simulink model "SNAP_Simulink_model_vtest"  (R2020b)
settings: Solver=VariableStepAuto  StartTime=0.0  StopTime=SNAP_sim_length  FixedStep=0.1  MaxStep=10  RelTol=1e-4  EnableMultiTasking=on
InitFcn:
  | SNAP_Simulink_Init_Function
undefined symbols (not defined in the file or in its folder): aeroCIP2006, EN_2BodyModel, EN_Aero, EN_GG, EN_Hyst, EN_Mag, initial_position, initial_velocity, magnitude, SNAP_Br, SNAP_Bs, SNAP_CONST_a3H0, SNAP_CONST_earth_mag_dipole, SNAP_CONST_G_earth, SNAP_CONST_m_earth, SNAP_CONST_mu0, SNAP_CONST_r_earth, SNAP_Hc, SNAP_init_rates, SNAP_JD, SNAP_magnets, SNAP_sat_inertia, SNAP_sat_mass, SNAP_starting_ECI2ECEF_dcm, SNAP_V_hyst, SNAPaero
libraries: vrlib x22, aerolibtransform2 x8, simulink x6, aerolibconvert2 x5, aerolibobsolete x1, aerolibanim x1
(part 1 of 2)
settings Model: Creator=Samir Rawashdeh  LastModifiedBy=colpari
settings DataIOCC: SaveFormat=Array  SignalLoggingSaveFormat=ModelDataLogs  ReturnWorkspaceOutputs=off
settings OptimizationCC: ExpressionDepthLimit=2147483647  LifeSpan=inf
settings DebuggingCC: UnderspecifiedInitializationDetection=Classic  MergeDetectMultiDrivingBlocksExec=none  SolverPrmCheckMsg=warning  MultiTaskCondExecSysMsg=warning  MultiTaskRateTransMsg=warning  SingleTaskRateTransMsg=warning  FcnCallInpInsideContextMsg=warning  StateNameClashWarn=warning  SFUnexpectedBacktrackingDiag=warning  SFNoUnconditionalDefaultTransitionDiag=warning  ArithmeticOperatorsInVariantConditions=warning
settings HardwareCC: ProdBitPerPointer=32  ProdBitPerSizeT=32  ProdBitPerPtrDiffT=32  ProdLargestAtomicFloat=None  ProdIntDivRoundTo=Undefined  ProdEndianess=Unspecified  ProdWordSize=32  ProdHWDeviceType=32-bit Generic
settings ModelReferenceCC: PropagateSignalLabelsOutOfModel=off
settings SFSimCC: SimUseLocalCustomCode=off  CustomCodeUndefinedFunction=UseInterfaceOnly
settings RTWCC: RTWUseLocalCustomCode=off
settings CodeAppCC: StateflowObjectComments=on
settings GRTTargetCC: TargetLangStandard=C89/C90 (ANSI)  CombineOutputUpdateFcns=off  GRTInterface=on
settings ConfigComp: CovMetricSettings=dw  CovSaveCumulativeToWorkspaceVar=on  CovSaveSingleToWorkspaceVar=on  CovExternalEMLEnable=off  CovSFcnEnable=off

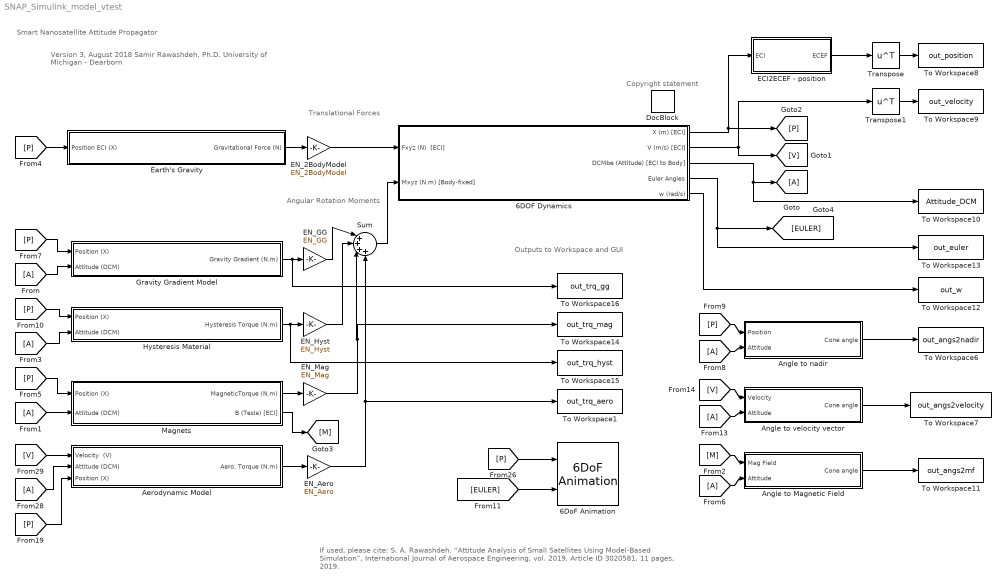
== system SNAP_Simulink_model_vtest ==
  note: If used, please cite:
      | S. A. Rawashdeh. “Attitude Analysis of Small Satellites Using Model-Based Simulation”, International Journal of
      |       Aerospace Engineering, vol. 2019, Article ID 3020581, 11 pages, 2019.
  note: Copyright statement
  note: Smart Nanosatellite Attitude Propagator
  note: Version 3, August 2018
      | Samir Rawashdeh, Ph.D.
      | University of Michigan - Dearborn
  note: Translational Forces
  note: Angular Rotation
      | Moments
  note: Outputs to Workspace and GUI
  "6DOF Dynamics " : Subsystem
  6DoF Animation : aerolibanim/6DoF Animation  u1=[-4000 4000 -2000 2000 -5000 -3000]  u2=10  u3=1000000*4  u4=[0 0 0]  u5=Fixed position  u6=[ 1 1 1 ] * 40000000  u7=15  u8=on
  Aerodynamic Model : Subsystem
  Angle to Magnetic Field : Subsystem
  Angle to nadir : Subsystem
  Angle to velocity vector : Subsystem
  DocBlock : simulink/Model-Wide Utilities/DocBlock  DocumentType=Text
      content=|
      | % See "help.txt" for documentation. More info in can be found at:
      | % sar-lab.net/snap
      | %
      | % -----------------------------------------------------------------------------
      | %   Copyright (c) 2010-2018 Samir A. Rawashdeh
      | %   Electrical and Computer Engineering
      | %   University of Michigan - Dearborn
      | %
      | %   All rights reserved.
      | %
      | %   Redistribution and use in source and binary forms, with or without
      | %   modification, are permitted provided that the following conditions are
      | %   met:
      | %
      | %       * Redistributions of source code must retain the above copyright
      | %         notice, this list of conditions and the following disclaimer.
      | %       * Redistributions in binary form must reproduce the above copyright
      | %         notice, this list of conditions and the following disclaimer in
      | %         the documentation and/or other materials provided with the distribution
      | %
      | %   THIS SOFTWARE IS PROVIDED BY THE COPYRIGHT HOLDERS AND CONTRIBUTORS "AS IS"
      | %   AND ANY EXPRESS OR IMPLIED WARRANTIES, INCLUDING, BUT NOT LIMITED TO, THE
      | %   IMPLIED WARRANTIES OF MERCHANTABILITY AND FITNESS FOR A PARTICULAR PURPOSE
      | %   ARE DISCLAIMED. IN NO EVENT SHALL THE COPYRIGHT OWNER OR CONTRIBUTORS BE
      | %   LIABLE FOR ANY DIRECT, INDIRECT, INCIDENTAL, SPECIAL, EXEMPLARY, OR
      | %   CONSEQUENTIAL DAMAGES (INCLUDING, BUT NOT LIMITED TO, PROCUREMENT OF
      | %   SUBSTITUTE GOODS OR SERVICES; LOSS OF USE, DATA, OR PROFITS; OR BUSINESS
      | %   INTERRUPTION) HOWEVER CAUSED AND ON ANY THEORY OF LIABILITY, WHETHER IN
      | %   CONTRACT, STRICT LIABILITY, OR TORT (INCLUDING NEGLIGENCE OR OTHERWISE)
      | %   ARISING IN ANY WAY OUT OF THE USE OF THIS SOFTWARE, EVEN IF ADVISED OF THE
      | %   POSSIBILITY OF SUCH DAMAGE.
      | %
      | % ----------------------------------------------------------------------------
  ECI2ECEF - position : Subsystem
  EN_2BodyModel : Gain  Gain=EN_2BodyModel
  "EN_Aero " : Gain  Gain=EN_Aero
  EN_GG : Gain  Gain=EN_GG
  EN_Hyst : Gain  Gain=EN_Hyst
  EN_Mag : Gain  Gain=EN_Mag
  Earth's Gravity : Subsystem
  Gravity Gradient Model : Subsystem
  Hysteresis Material : Subsystem
  Magnets : Subsystem
  Sum : Sum  Inputs=|++++
  To Workspace1 : ToWorkspace  VariableName=out_trq_aero  SaveFormat=Structure With Time  SampleTime=-1
  To Workspace10 : ToWorkspace  VariableName=Attitude_DCM  SaveFormat=Structure With Time  SampleTime=-1
  To Workspace11 : ToWorkspace  VariableName=out_angs2mf  SaveFormat=Structure With Time  SampleTime=-1
  To Workspace12 : ToWorkspace  VariableName=out_w  SaveFormat=Structure With Time  SampleTime=-1
  To Workspace13 : ToWorkspace  VariableName=out_euler  SaveFormat=Structure With Time  SampleTime=-1
  To Workspace14 : ToWorkspace  VariableName=out_trq_mag  SaveFormat=Structure With Time  SampleTime=-1
  To Workspace15 : ToWorkspace  VariableName=out_trq_hyst  SaveFormat=Structure With Time  SampleTime=-1
  To Workspace16 : ToWorkspace  VariableName=out_trq_gg  SaveFormat=Structure With Time  SampleTime=-1
  To Workspace6 : ToWorkspace  VariableName=out_angs2nadir  SaveFormat=Structure With Time  SampleTime=-1
  To Workspace7 : ToWorkspace  VariableName=out_angs2velocity  SaveFormat=Structure With Time  SampleTime=-1
  To Workspace8 : ToWorkspace  VariableName=out_position  SaveFormat=Structure With Time  SampleTime=-1
  To Workspace9 : ToWorkspace  VariableName=out_velocity  SaveFormat=Structure With Time  SampleTime=-1
  Transpose : Math  Operator=transpose  SignedPower=on  SaturateOnIntegerOverflow=on
  Transpose1 : Math  Operator=transpose  SignedPower=on  SaturateOnIntegerOverflow=on
  wires:
  Transpose/1 -> To Workspace8/1
  Transpose1/1 -> To Workspace9/1
  "6DOF Dynamics "/3(DCMbe (Attitude) [ECI to Body]) -> To Workspace10/1, [A]
  "6DOF Dynamics "/4(Euler Angles) -> [EULER], To Workspace13/1
  "6DOF Dynamics "/5(w (rad/s)) -> To Workspace12/1
  Gravity Gradient Model/1(Gravity Gradient (N.m)) -> To Workspace16/1, EN_GG/1
  Hysteresis Material/1(Hysteresis Torque (N.m)) -> EN_Hyst/1, To Workspace15/1
  EN_Mag/1 -> Sum/3, To Workspace14/1
  Angle to nadir/1(Cone angle) -> To Workspace6/1
  Angle to velocity vector/1(Cone angle) -> To Workspace7/1
  [P] -> Earth's Gravity/1(Position ECI (X))
  "6DOF Dynamics "/1(X (m) [ECI]) -> ECI2ECEF - position/1(ECI), [P]
  "6DOF Dynamics "/2(V (m/s) [ECI]) -> Transpose1/1, [V]
  [P] -> Gravity Gradient Model/1(Position (X))
  [A] -> Gravity Gradient Model/2(Attitude (DCM))
  [P] -> Magnets/1(Position (X))
  [A] -> Magnets/2(Attitude (DCM))
  Magnets/1(MagneticTorque (N.m)) -> EN_Mag/1
  [A] -> Angle to nadir/2(Attitude)
  [P] -> Angle to nadir/1(Position)
  [A] -> Angle to velocity vector/2(Attitude)
  [V] -> Angle to velocity vector/1(Velocity)
  ECI2ECEF - position/1(ECEF) -> Transpose/1
  Magnets/2(B (Tesla) [ECI]) -> [M]
  Earth's Gravity/1(Gravitational Force (N)) -> EN_2BodyModel/1
  [A] -> Angle to Magnetic Field/2(Attitude)
  Angle to Magnetic Field/1(Cone angle) -> To Workspace11/1
  [M] -> Angle to Magnetic Field/1(Mag Field)
  EN_GG/1 -> Sum/1
  EN_Hyst/1 -> Sum/2
  [V] -> Aerodynamic Model/1(Velocity  (V))
  [A] -> Aerodynamic Model/2(Attitude (DCM))
  [P] -> Aerodynamic Model/3(Position (X))
  [P] -> 6DoF Animation/1
  EN_2BodyModel/1 -> "6DOF Dynamics "/1(Fxyz (N)  [ECI])
  Sum/1 -> "6DOF Dynamics "/2(Mxyz (N.m) [Body-fixed])
  [P] -> Hysteresis Material/1(Position (X))
  [A] -> Hysteresis Material/2(Attitude (DCM))
  Aerodynamic Model/1(Aero. Torque (N.m)) -> "EN_Aero "/1
  "EN_Aero "/1 -> Sum/4, To Workspace1/1
  [EULER] -> 6DoF Animation/2

== system SNAP_Simulink_model_vtest/6DOF Dynamics  ==
  Fxyz (N)  [ECI] : Inport
  Mxyz (N.m) [Body-fixed] : Inport  Port=2
  Rotations - 6DoF (Quaternion) : aerolibobsolete/6DoF (Euler Angles)  units=Metric (MKS)  mtype=Fixed  rep=Quaternion  xme_0=[0 0 0] % not used  Vm_0=[0 0 0] % not used  eul_0=[0 0 0] %[0 pi/1.1 0]  pm_0=SNAP_init_rates %(ones(1,3)*0.5-rand(1,3) )* 2 * .3 *pi/180;  mass_0=SNAP_sat_mass  mass_e=0  mass_f=0  inertia=SNAP_sat_inertia  inertia_e=eye(3)  inertia_f=eye(3)  k_quat=1.0
      settings: SourceProductBaseCode=AE
  Terminator{,1..3,5} (5 alike) : Terminator
  Translation : Subsystem
  zero : Constant  Value=[0 0 0]
  X (m) [ECI] : Outport
  V (m/s) [ECI] : Outport  Port=2
  DCMbe (Attitude) [ECI to Body] : Outport  Port=3
  Euler Angles : Outport  Port=4
  w (rad/s) : Outport  Port=5
  wires:
  Rotations - 6DoF (Quaternion)/2 -> Terminator/1
  Rotations - 6DoF (Quaternion)/1 -> Terminator2/1
  Rotations - 6DoF (Quaternion)/5 -> Terminator1/1
  Translation/1(Xe(m) (ECI)) -> X (m) [ECI]/1
  Translation/2(Ve(m/s) (ECI)) -> V (m/s) [ECI]/1
  Rotations - 6DoF (Quaternion)/6 -> w (rad/s)/1
  Rotations - 6DoF (Quaternion)/8 -> Terminator5/1
  Rotations - 6DoF (Quaternion)/7 -> Terminator3/1
  zero/1 -> Rotations - 6DoF (Quaternion)/1
  Fxyz (N)  [ECI]/1 -> Translation/1(Fxyz (N) (inECI))
  Mxyz (N.m) [Body-fixed]/1 -> Rotations - 6DoF (Quaternion)/2
  Rotations - 6DoF (Quaternion)/3 -> Euler Angles/1
  Rotations - 6DoF (Quaternion)/4 -> DCMbe (Attitude) [ECI to Body]/1

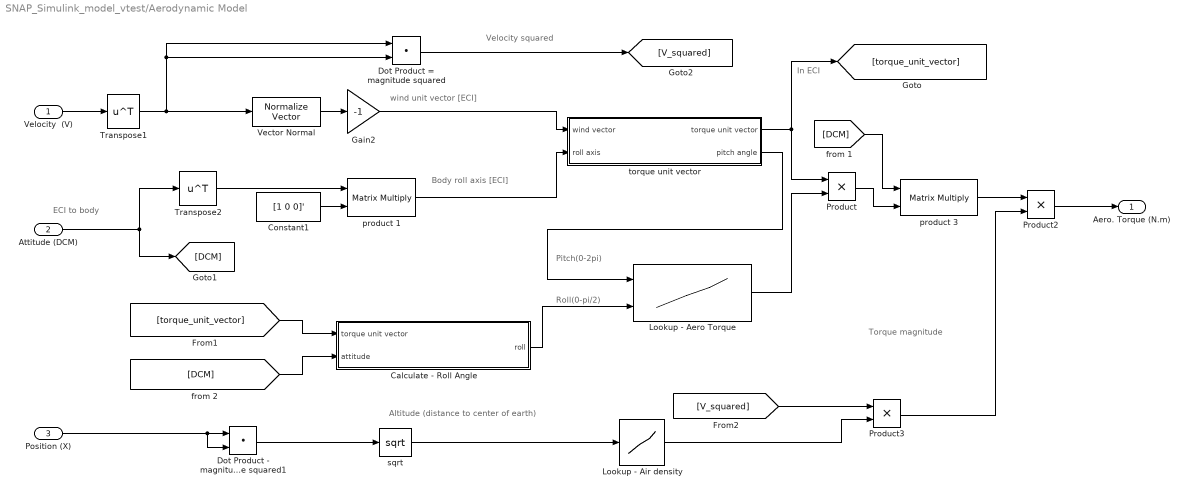
== system SNAP_Simulink_model_vtest/Aerodynamic Model ==
  note: Pitch(0-2pi)
  note: wind unit vector [ECI]
  note: Torque magnitude
  note: Body roll axis [ECI]
  note: In ECI
  note: ECI to body
  note: Velocity squared
  note: Roll(0-pi/2)
  note: Altitude (distance to center of earth)
  Velocity  (V) : Inport
  Attitude (DCM) : Inport  Port=2
  Position (X) : Inport  Port=3
  Calculate - Roll Angle : Subsystem
  Constant1 : Constant  Value=[1 0 0]'
  Dot Product - magnitude squared1 : DotProduct  InputSameDT=on  OutDataTypeStr=Inherit: Inherit via internal rule
  Dot Product = magnitude squared : DotProduct  InputSameDT=on  OutDataTypeStr=Inherit: Inherit via internal rule
  Gain2 : Gain  Gain=-1
  Lookup - Aero Torque : Lookup2D  RowIndex=SNAPaero.pitch  ColumnIndex=SNAPaero.roll  Table=SNAPaero.T
  Lookup - Air density : Lookup  InputValues=SNAPaero.alt_range*1000 + SNAP_CONST_r_earth  Table=SNAPaero.av_density_vs_alt
  Product : Product  RndMeth=Zero
  Product2 : Product  RndMeth=Zero
  Product3 : Product  RndMeth=Zero
  Transpose1 : Math  Operator=transpose  SignedPower=on  SaturateOnIntegerOverflow=on
  Transpose2 : Math  Operator=transpose  SignedPower=on  SaturateOnIntegerOverflow=on
  Vector Normal : vrlib/Utilities/Normalize Vector  maxzero=0
  product 1 : Product  Multiplication=Matrix(*)  RndMeth=Zero
  product 3 : Product  Multiplication=Matrix(*)  RndMeth=Zero
  sqrt : Math  Operator=sqrt  SignedPower=on  SaturateOnIntegerOverflow=on
  torque unit vector : Subsystem
  Aero. Torque (N.m) : Outport
  wires:
  Velocity  (V)/1 -> Transpose1/1
  Dot Product = magnitude squared/1 -> [V_squared]
  Vector Normal/1 -> Gain2/1
  Gain2/1 -> torque unit vector/1(wind vector)
  product 1/1 -> torque unit vector/2(roll axis)
  torque unit vector/1(torque unit vector) -> Product/1, [torque_unit_vector]
  Lookup - Aero Torque/1 -> Product/2
  [DCM] -> product 3/1
  Transpose1/1 -> Vector Normal/1, Dot Product = magnitude squared/2, Dot Product = magnitude squared/1
  Constant1/1 -> product 1/2
  Attitude (DCM)/1 -> [DCM], Transpose2/1
  Product/1 -> product 3/2
  Calculate - Roll Angle/1(roll) -> Lookup - Aero Torque/2
  torque unit vector/2(pitch angle) -> Lookup - Aero Torque/1
  Transpose2/1 -> product 1/1
  [torque_unit_vector] -> Calculate - Roll Angle/1(torque unit vector)
  [DCM] -> Calculate - Roll Angle/2(attitude)
  Position (X)/1 -> Dot Product - magnitude squared1/1, Dot Product - magnitude squared1/2
  Dot Product - magnitude squared1/1 -> sqrt/1
  sqrt/1 -> Lookup - Air density/1
  Lookup - Air density/1 -> Product3/2
  Product3/1 -> Product2/2
  [V_squared] -> Product3/1
  Product2/1 -> Aero. Torque (N.m)/1
  product 3/1 -> Product2/1

== system SNAP_Simulink_model_vtest/Angle to Magnetic Field ==
  note: velocity vector
  Mag Field : Inport
  Attitude : Inport  Port=2
  Normalize Vector : vrlib/Utilities/Normalize Vector  maxzero=0
  cosines to body axes : Subsystem
  Cone angle : Outport
  wires:
  Mag Field/1 -> Normalize Vector/1
  Attitude/1 -> cosines to body axes/2(Attitude)
  cosines to body axes/1(Cone Angles) -> Cone angle/1
  Normalize Vector/1 -> cosines to body axes/1(Reference Vector)

== system SNAP_Simulink_model_vtest/Angle to nadir ==
  note: vector from satellite to earth (nadir)
  Position : Inport
  Attitude : Inport  Port=2
  Gain2 : Gain  Gain=-1
  Normalize Vector : vrlib/Utilities/Normalize Vector  maxzero=0
  cosines to body axes : Subsystem
  Cone angle : Outport
  wires:
  Normalize Vector/1 -> Gain2/1
  Position/1 -> Normalize Vector/1
  cosines to body axes/1(Cone Angles) -> Cone angle/1
  Gain2/1 -> cosines to body axes/1(Reference Vector)
  Attitude/1 -> cosines to body axes/2(Attitude)

== system SNAP_Simulink_model_vtest/Angle to velocity vector ==
  note: velocity vector
  Velocity : Inport
  Attitude : Inport  Port=2
  Normalize Vector : vrlib/Utilities/Normalize Vector  maxzero=0
  cosines to body axes : Subsystem
  Cone angle : Outport
  wires:
  Velocity/1 -> Normalize Vector/1
  Attitude/1 -> cosines to body axes/2(Attitude)
  cosines to body axes/1(Cone Angles) -> Cone angle/1
  Normalize Vector/1 -> cosines to body axes/1(Reference Vector)

== system SNAP_Simulink_model_vtest/ECI2ECEF - position ==
  ECI : Inport
  Constant : Constant  Value=[0 0]
  Constant1 : Constant  Commented=on  Value=SNAP_JD
  Constant2 : Constant  Value=SNAP_starting_ECI2ECEF_dcm
  Direction Cosine Matrix ECI to ECEF1 : Subsystem  Commented=on  AncestorBlock=aerolibtransform2/Direction Cosine Matrix ECI to ECEF  mask{red=IAU-2000/2006, deltaT=Sec, errorflag=Error, extraparamflag=off}
      mask prompts: red "aeroblks:aeroblktransform:blockDCMECItoECEFParamReduction"; deltaT "aeroblks:aeroblktransform:blockDCMECItoECEFParamTimeincrement"; errorflag "aeroblks:aeroblktransform:blockDCMECItoECEFParamActionforoutofrangeinput"; extraparamflag "aeroblks:aeroblktransform:blockDCMECItoECEFParamHigheraccuracyparameters"
      settings: AttributesFormatString=%<red>
      mask TypeOptions red: aeroblks:aeroblktransform:blockDCMECItoECEFParamComboIAU76FK5 | aeroblks:aeroblktransform:blockDCMECItoECEFParamComboIAU20002006
      mask TypeOptions deltaT: aeroblks:aeroblktransform:blockDCMECItoECEFParamComboNone | aeroblks:aeroblktransform:blockDCMECItoECEFParamComboDay | aeroblks:aeroblktransform:blockDCMECItoECEFParamComboHour | aeroblks:aeroblktransform:blockDCMECItoECEFParamComboMin | aeroblks:aeroblktransform:blockDCMECItoECEFParamComboSec
      mask TypeOptions errorflag: aeroblks:aeroblktransform:blockDCMECItoECEFParamComboNone | aeroblks:aeroblktransform:blockDCMECItoECEFParamComboWarning | aeroblks:aeroblktransform:blockDCMECItoECEFParamComboError
      mask Display:
      | port_label('output',1,'DCM_{fi}','texmode','on')
      | port_label('input',1,'JD')
  Gain : Gain  Gain=-1
  Mux : Mux  Inputs=2
  Ramp1 : simulink/Sources/Ramp  slope="7.292115856e-5   %2*pi/(24*60*60)  %radians/second (one rotation per day )"  start=0  X0=0
  Rotation Angles to Direction Cosine Matrix : aerolibtransform2/Rotation Angles to Direction Cosine Matrix  rotationOrder=ZYX
      settings: SourceProductBaseCode=AE
  product 1 : Product  Multiplication=Matrix(*)  RndMeth=Zero
  product 2 : Product  Multiplication=Matrix(*)  RndMeth=Zero
  ECEF : Outport
  wires:
  product 2/1 -> ECEF/1
  ECI/1 -> product 2/1
  Constant1/1 -> Direction Cosine Matrix ECI to ECEF1/1(JD)
  Ramp1/1 -> Gain/1
  Gain/1 -> Mux/1
  Mux/1 -> Rotation Angles to Direction Cosine Matrix/1
  Constant/1 -> Mux/2
  product 1/1 -> product 2/2
  Rotation Angles to Direction Cosine Matrix/1 -> product 1/2
  Constant2/1 -> product 1/1

== system SNAP_Simulink_model_vtest/Earth's Gravity ==
  note: Gravitational
      | acceleration vector
  note: magnitude of acceleration due to gravity
  note: Unit vector towards Nadir
  note: a_gravity = G*m/r^2
  Position ECI (X) : Inport
  Constant : Constant  Value=SNAP_CONST_r_earth
  Divide : Product  Inputs=*/
  Gain1 : Gain  Gain=-1
  Gain2 : Gain  Gain=SNAP_sat_mass
  Gravitational Constant : Constant  Value=SNAP_CONST_m_earth*SNAP_CONST_G_earth
  Math Function : Math  Operator=sqrt  SignedPower=on  SaturateOnIntegerOverflow=on
  Product : Product  RndMeth=Zero
  Scope4 : Scope
  Sum : Sum  Inputs=|+-
  Vector Dot Product = magnitude squared : DotProduct  InputSameDT=on  OutDataTypeStr=Inherit: Inherit via internal rule
  Vector Normal : vrlib/Utilities/Normalize Vector  maxzero=0
  Gravitational Force (N) : Outport
  wires:
  Position ECI (X)/1 -> Vector Normal/1, Vector Dot Product = magnitude squared/1, Vector Dot Product = magnitude squared/2
  Vector Normal/1 -> Gain1/1
  Gain1/1 -> Product/1
  Product/1 -> Gain2/1
  Vector Dot Product = magnitude squared/1 -> Divide/2, Math Function/1
  Divide/1 -> Product/2
  Gravitational Constant/1 -> Divide/1
  Gain2/1 -> Gravitational Force (N)/1
  Math Function/1 -> Sum/1
  Sum/1 -> Scope4/1
  Constant/1 -> Sum/2

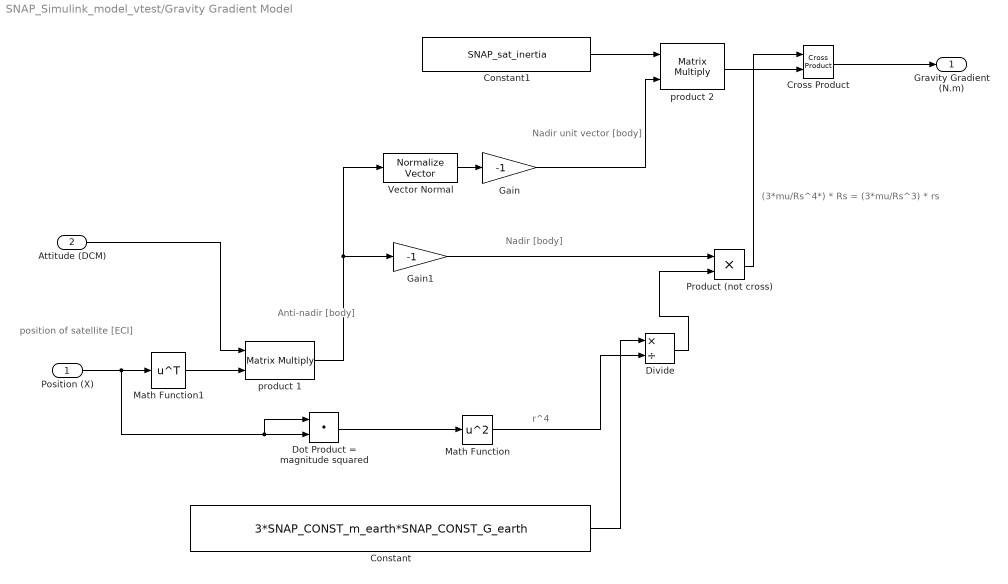
== system SNAP_Simulink_model_vtest/Gravity Gradient Model ==
  note: (3*mu/Rs^4*) * Rs = (3*mu/Rs^3) * rs
  note: Nadir [body]
  note: position of satellite [ECI]
  note: Nadir unit vector
      | [body]
  note: Anti-nadir [body]
  note: r^4
  Position (X) : Inport
  Attitude (DCM) : Inport  Port=2
  Constant : Constant  Value=3*SNAP_CONST_m_earth*SNAP_CONST_G_earth
  Constant1 : Constant  Value=SNAP_sat_inertia
  Cross Product : vrlib/Utilities/Cross Product
  Divide : Product  Inputs=*/
  Dot Product = magnitude squared : DotProduct  InputSameDT=on  OutDataTypeStr=Inherit: Inherit via internal rule
  Gain : Gain  Gain=-1
  Gain1 : Gain  Gain=-1
  Math Function : Math  Operator=square  SignedPower=on  SaturateOnIntegerOverflow=on
  Math Function1 : Math  Operator=transpose  SignedPower=on  SaturateOnIntegerOverflow=on
  Product (not cross) : Product  RndMeth=Zero
  Vector Normal : vrlib/Utilities/Normalize Vector  maxzero=0
  product 1 : Product  Multiplication=Matrix(*)  RndMeth=Zero
  product 2 : Product  Multiplication=Matrix(*)  RndMeth=Zero
  Gravity Gradient (N.m) : Outport
  wires:
  Product (not cross)/1 -> Cross Product/1
  Divide/1 -> Product (not cross)/2
  Constant/1 -> Divide/1
  Math Function/1 -> Divide/2
  Vector Normal/1 -> Gain/1
  Cross Product/1 -> Gravity Gradient (N.m)/1
  Dot Product = magnitude squared/1 -> Math Function/1
  Gain/1 -> product 2/2
  product 2/1 -> Cross Product/2
  Constant1/1 -> product 2/1
  Position (X)/1 -> Dot Product = magnitude squared/2, Dot Product = magnitude squared/1, Math Function1/1
  Attitude (DCM)/1 -> product 1/1
  product 1/1 -> Vector Normal/1, Gain1/1
  Gain1/1 -> Product (not cross)/1
  Math Function1/1 -> product 1/2

== system SNAP_Simulink_model_vtest/Hysteresis Material ==
  note: ECI to Body
  note: T = m X B
  note: B_earth
  note: B_earth [body]
  note: m [body]
  Position (X) : Inport
  Attitude (DCM) : Inport  Port=2
  Cross Product : vrlib/Utilities/Cross Product
  Eearth L-Shell Magnetic Model : Subsystem
  Gain : Gain  Gain=1/SNAP_CONST_mu0
  Hysteresis Curve Model : Subsystem
  Product : Product  Multiplication=Matrix(*)  RndMeth=Zero
  Transpose : Math  Operator=transpose  SignedPower=on  SaturateOnIntegerOverflow=on
  m = B*V/mu0 : Product  RndMeth=Zero
  zero : Constant  Value=SNAP_V_hyst/SNAP_CONST_mu0
  Hysteresis Torque (N.m) : Outport
  wires:
  Product/1 -> Gain/1, Cross Product/2
  Cross Product/1 -> Hysteresis Torque (N.m)/1
  zero/1 -> m = B*V/mu0/2
  m = B*V/mu0/1 -> Cross Product/1
  Attitude (DCM)/1 -> Product/1
  Eearth L-Shell Magnetic Model/1(B (Tesla) in ECI) -> Transpose/1
  Transpose/1 -> Product/2
  Gain/1 -> Hysteresis Curve Model/1(H)
  Hysteresis Curve Model/1(B) -> m = B*V/mu0/1
  Position (X)/1 -> Eearth L-Shell Magnetic Model/1(Position in ECI)

== system SNAP_Simulink_model_vtest/Magnets ==
  note: T = m X B
  note: B_earth [body]
  note: ECI to Body
  Position (X) : Inport
  Attitude (DCM) : Inport  Port=2
  Cross Product : vrlib/Utilities/Cross Product
  Eearth L-Shell Magnetic Model : Subsystem
  Product : Product  Multiplication=Matrix(*)  RndMeth=Zero
  Transpose : Math  Operator=transpose  SignedPower=on  SaturateOnIntegerOverflow=on
  constant : Constant  Value=SNAP_magnets
  MagneticTorque (N.m) : Outport
  B (Tesla) [ECI] : Outport  Port=2
  wires:
  Position (X)/1 -> Eearth L-Shell Magnetic Model/1(Position in ECI)
  Product/1 -> Cross Product/2
  Cross Product/1 -> MagneticTorque (N.m)/1
  constant/1 -> Cross Product/1
  Attitude (DCM)/1 -> Product/1
  Eearth L-Shell Magnetic Model/1(B (Tesla) in ECI) -> Transpose/1, B (Tesla) [ECI]/1
  Transpose/1 -> Product/2

== system SNAP_Simulink_model_vtest/6DOF Dynamics /Translation ==
  note: Force
  note: Acceleration
  note: Velocity
  note: Position
  Fxyz (N) (inECI) : Inport
  Gain : Gain  Gain=1/SNAP_sat_mass
  Integrator : Integrator  InitialCondition=initial_velocity
  Integrator1 : Integrator  InitialCondition=initial_position
  Xe(m) (ECI) : Outport
  Ve(m/s) (ECI) : Outport  Port=2
  wires:
  Fxyz (N) (inECI)/1 -> Gain/1
  Gain/1 -> Integrator/1
  Integrator/1 -> Integrator1/1, Ve(m/s) (ECI)/1
  Integrator1/1 -> Xe(m) (ECI)/1

== system SNAP_Simulink_model_vtest/Aerodynamic Model/Calculate - Roll Angle ==
  note: pitch axis in ECI
  note: Roll(0-pi/2)
  torque unit vector : Inport
  attitude : Inport  Port=2
  Constant2 : Constant  Value=[0 1 0]'
  Constant3 : Constant  Value=pi/2
  Dot Product : DotProduct  InputSameDT=on  OutDataTypeStr=Inherit: Inherit via internal rule
  Modulus : Math  Operator=mod  SignedPower=on  SaturateOnIntegerOverflow=on
  Trigonometric Function1 : Trigonometry  Operator=acos
  product 2 : Product  Multiplication=Matrix(*)  RndMeth=Zero
  roll : Outport
  wires:
  torque unit vector/1 -> Dot Product/1
  product 2/1 -> Dot Product/2
  Dot Product/1 -> Trigonometric Function1/1
  Trigonometric Function1/1 -> Modulus/1
  Constant3/1 -> Modulus/2
  Modulus/1 -> roll/1
  Constant2/1 -> product 2/2
  attitude/1 -> product 2/1

== system SNAP_Simulink_model_vtest/Aerodynamic Model/torque unit vector ==
  wind vector : Inport
  roll axis : Inport  Port=2
  Cross Product : vrlib/Utilities/Cross Product
  Dot Product : DotProduct  InputSameDT=on  OutDataTypeStr=Inherit: Inherit via internal rule
  Normalize Vector : vrlib/Utilities/Normalize Vector  maxzero=0
  Trigonometric Function2 : Trigonometry  Operator=acos
  torque unit vector : Outport
  pitch angle : Outport  Port=2
  wires:
  Normalize Vector/1 -> torque unit vector/1
  Cross Product/1 -> Normalize Vector/1
  wind vector/1 -> Cross Product/1, Dot Product/1
  roll axis/1 -> Cross Product/2, Dot Product/2
  Dot Product/1 -> Trigonometric Function2/1
  Trigonometric Function2/1 -> pitch angle/1

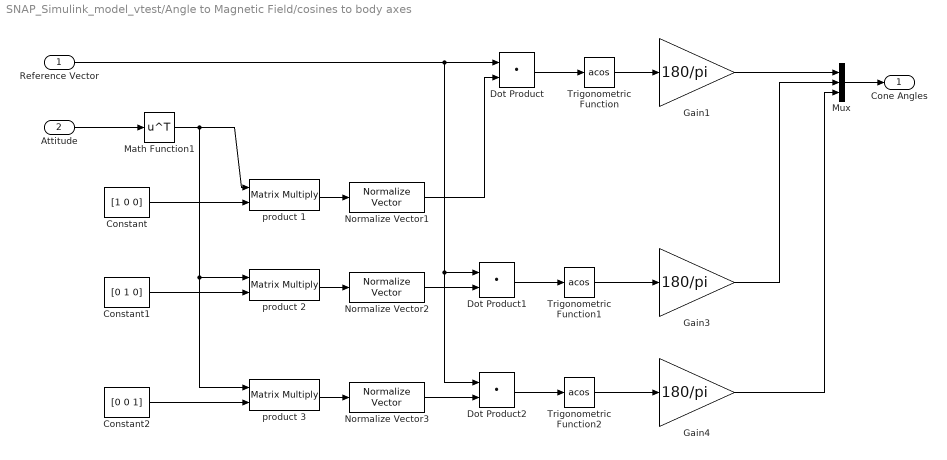
== system SNAP_Simulink_model_vtest/Angle to Magnetic Field/cosines to body axes ==
  Reference Vector : Inport
  Attitude : Inport  Port=2
  Constant : Constant  Value=[1 0 0]
  Constant1 : Constant  Value=[0 1 0]
  Constant2 : Constant  Value=[0 0 1]
  Dot Product : DotProduct  InputSameDT=on  OutDataTypeStr=Inherit: Inherit via internal rule
  Dot Product1 : DotProduct  InputSameDT=on  OutDataTypeStr=Inherit: Inherit via internal rule
  Dot Product2 : DotProduct  InputSameDT=on  OutDataTypeStr=Inherit: Inherit via internal rule
  Gain1 : Gain  Gain=180/pi
  Gain3 : Gain  Gain=180/pi
  Gain4 : Gain  Gain=180/pi
  Math Function1 : Math  Operator=transpose  SignedPower=on  SaturateOnIntegerOverflow=on
  Mux : Mux  Inputs=3
  Normalize Vector1 : vrlib/Utilities/Normalize Vector  maxzero=0
  Normalize Vector2 : vrlib/Utilities/Normalize Vector  maxzero=0
  Normalize Vector3 : vrlib/Utilities/Normalize Vector  maxzero=0
  Trigonometric Function : Trigonometry  Operator=acos
  Trigonometric Function1 : Trigonometry  Operator=acos
  Trigonometric Function2 : Trigonometry  Operator=acos
  product 1 : Product  Multiplication=Matrix(*)  RndMeth=Zero
  product 2 : Product  Multiplication=Matrix(*)  RndMeth=Zero
  product 3 : Product  Multiplication=Matrix(*)  RndMeth=Zero
  Cone Angles : Outport
  wires:
  product 1/1 -> Normalize Vector1/1
  Reference Vector/1 -> Dot Product/1, Dot Product1/1, Dot Product2/1
  Normalize Vector1/1 -> Dot Product/2
  Dot Product/1 -> Trigonometric Function/1
  Trigonometric Function/1 -> Gain1/1
  Attitude/1 -> Math Function1/1
  Constant/1 -> product 1/2
  Math Function1/1 -> product 1/1, product 2/1, product 3/1
  Mux/1 -> Cone Angles/1
  Gain1/1 -> Mux/1
  Dot Product1/1 -> Trigonometric Function1/1
  Trigonometric Function1/1 -> Gain3/1
  Dot Product2/1 -> Trigonometric Function2/1
  Trigonometric Function2/1 -> Gain4/1
  Gain3/1 -> Mux/2
  Gain4/1 -> Mux/3
  product 2/1 -> Normalize Vector2/1
  Constant1/1 -> product 2/2
  product 3/1 -> Normalize Vector3/1
  Constant2/1 -> product 3/2
  Normalize Vector2/1 -> Dot Product1/2
  Normalize Vector3/1 -> Dot Product2/2

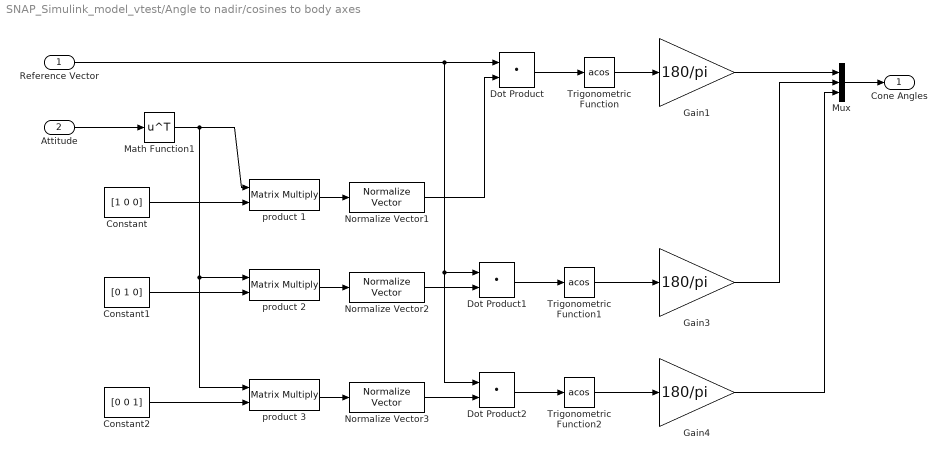
== system SNAP_Simulink_model_vtest/Angle to nadir/cosines to body axes ==
  Reference Vector : Inport
  Attitude : Inport  Port=2
  Constant : Constant  Value=[1 0 0]
  Constant1 : Constant  Value=[0 1 0]
  Constant2 : Constant  Value=[0 0 1]
  Dot Product : DotProduct  InputSameDT=on  OutDataTypeStr=Inherit: Inherit via internal rule
  Dot Product1 : DotProduct  InputSameDT=on  OutDataTypeStr=Inherit: Inherit via internal rule
  Dot Product2 : DotProduct  InputSameDT=on  OutDataTypeStr=Inherit: Inherit via internal rule
  Gain1 : Gain  Gain=180/pi
  Gain3 : Gain  Gain=180/pi
  Gain4 : Gain  Gain=180/pi
  Math Function1 : Math  Operator=transpose  SignedPower=on  SaturateOnIntegerOverflow=on
  Mux : Mux  Inputs=3
  Normalize Vector1 : vrlib/Utilities/Normalize Vector  maxzero=0
  Normalize Vector2 : vrlib/Utilities/Normalize Vector  maxzero=0
  Normalize Vector3 : vrlib/Utilities/Normalize Vector  maxzero=0
  Trigonometric Function : Trigonometry  Operator=acos
  Trigonometric Function1 : Trigonometry  Operator=acos
  Trigonometric Function2 : Trigonometry  Operator=acos
  product 1 : Product  Multiplication=Matrix(*)  RndMeth=Zero
  product 2 : Product  Multiplication=Matrix(*)  RndMeth=Zero
  product 3 : Product  Multiplication=Matrix(*)  RndMeth=Zero
  Cone Angles : Outport
  wires:
  product 1/1 -> Normalize Vector1/1
  Reference Vector/1 -> Dot Product/1, Dot Product1/1, Dot Product2/1
  Normalize Vector1/1 -> Dot Product/2
  Dot Product/1 -> Trigonometric Function/1
  Trigonometric Function/1 -> Gain1/1
  Attitude/1 -> Math Function1/1
  Constant/1 -> product 1/2
  Math Function1/1 -> product 1/1, product 2/1, product 3/1
  Mux/1 -> Cone Angles/1
  Gain1/1 -> Mux/1
  Dot Product1/1 -> Trigonometric Function1/1
  Trigonometric Function1/1 -> Gain3/1
  Dot Product2/1 -> Trigonometric Function2/1
  Trigonometric Function2/1 -> Gain4/1
  Gain3/1 -> Mux/2
  Gain4/1 -> Mux/3
  product 2/1 -> Normalize Vector2/1
  Constant1/1 -> product 2/2
  product 3/1 -> Normalize Vector3/1
  Constant2/1 -> product 3/2
  Normalize Vector2/1 -> Dot Product1/2
  Normalize Vector3/1 -> Dot Product2/2

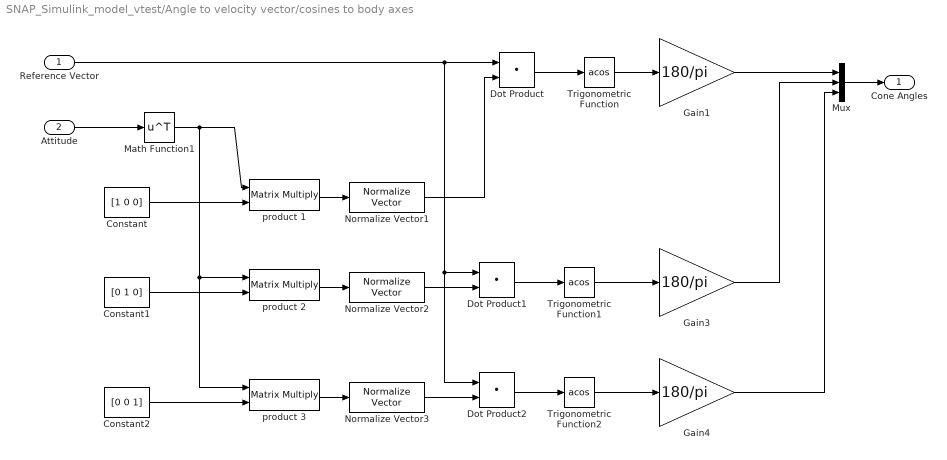
== system SNAP_Simulink_model_vtest/Angle to velocity vector/cosines to body axes ==
  Reference Vector : Inport
  Attitude : Inport  Port=2
  Constant : Constant  Value=[1 0 0]
  Constant1 : Constant  Value=[0 1 0]
  Constant2 : Constant  Value=[0 0 1]
  Dot Product : DotProduct  InputSameDT=on  OutDataTypeStr=Inherit: Inherit via internal rule
  Dot Product1 : DotProduct  InputSameDT=on  OutDataTypeStr=Inherit: Inherit via internal rule
  Dot Product2 : DotProduct  InputSameDT=on  OutDataTypeStr=Inherit: Inherit via internal rule
  Gain1 : Gain  Gain=180/pi
  Gain3 : Gain  Gain=180/pi
  Gain4 : Gain  Gain=180/pi
  Math Function1 : Math  Operator=transpose  SignedPower=on  SaturateOnIntegerOverflow=on
  Mux : Mux  Inputs=3
  Normalize Vector1 : vrlib/Utilities/Normalize Vector  maxzero=0
  Normalize Vector2 : vrlib/Utilities/Normalize Vector  maxzero=0
  Normalize Vector3 : vrlib/Utilities/Normalize Vector  maxzero=0
  Trigonometric Function : Trigonometry  Operator=acos
  Trigonometric Function1 : Trigonometry  Operator=acos
  Trigonometric Function2 : Trigonometry  Operator=acos
  product 1 : Product  Multiplication=Matrix(*)  RndMeth=Zero
  product 2 : Product  Multiplication=Matrix(*)  RndMeth=Zero
  product 3 : Product  Multiplication=Matrix(*)  RndMeth=Zero
  Cone Angles : Outport
  wires:
  product 1/1 -> Normalize Vector1/1
  Reference Vector/1 -> Dot Product/1, Dot Product1/1, Dot Product2/1
  Normalize Vector1/1 -> Dot Product/2
  Dot Product/1 -> Trigonometric Function/1
  Trigonometric Function/1 -> Gain1/1
  Attitude/1 -> Math Function1/1
  Constant/1 -> product 1/2
  Math Function1/1 -> product 1/1, product 2/1, product 3/1
  Mux/1 -> Cone Angles/1
  Gain1/1 -> Mux/1
  Dot Product1/1 -> Trigonometric Function1/1
  Trigonometric Function1/1 -> Gain3/1
  Dot Product2/1 -> Trigonometric Function2/1
  Trigonometric Function2/1 -> Gain4/1
  Gain3/1 -> Mux/2
  Gain4/1 -> Mux/3
  product 2/1 -> Normalize Vector2/1
  Constant1/1 -> product 2/2
  product 3/1 -> Normalize Vector3/1
  Constant2/1 -> product 3/2
  Normalize Vector2/1 -> Dot Product1/2
  Normalize Vector3/1 -> Dot Product2/2

== system SNAP_Simulink_model_vtest/ECI2ECEF - position/Direction Cosine Matrix ECI to ECEF1 ==
  JD : Inport  OutMin=0  PortDimensions=1
  AddParam : Constant  Value="[0  0]"
  Common Time Calculation : Subsystem
  IAUReduction : Subsystem  AncestorBlock=aerolibtransform2sys/IAU20002006  mask{deltaT=Sec, Sdata=0, XYdata=0}
      mask prompts: deltaT "Time Increment"
      mask init:
      | load aeroCIP2006.mat
      mask TypeOptions deltaT: None | Day | Hour | Min | Sec
  PolarMotion : Constant  Value="[0  0]"
  deltaAT : Constant  Value=[0]
  deltaUT1 : Constant  Value=[0]
  DCM : Outport
  wires:
  deltaAT/1 -> Common Time Calculation/3(deltaAT)
  deltaUT1/1 -> Common Time Calculation/2(deltaUT1)
  PolarMotion/1 -> IAUReduction/6("[xp,yp]")
  Common Time Calculation/3(jdTT) -> IAUReduction/5(jdTT)
  AddParam/1 -> IAUReduction/1("[dX,dY]")
  Common Time Calculation/1(tTT) -> IAUReduction/3(tTT)
  Common Time Calculation/2(ssUT) -> IAUReduction/4(ssUT)
  IAUReduction/1(DCM) -> DCM/1
  JD/1 -> IAUReduction/2("JD "), Common Time Calculation/1(JD)

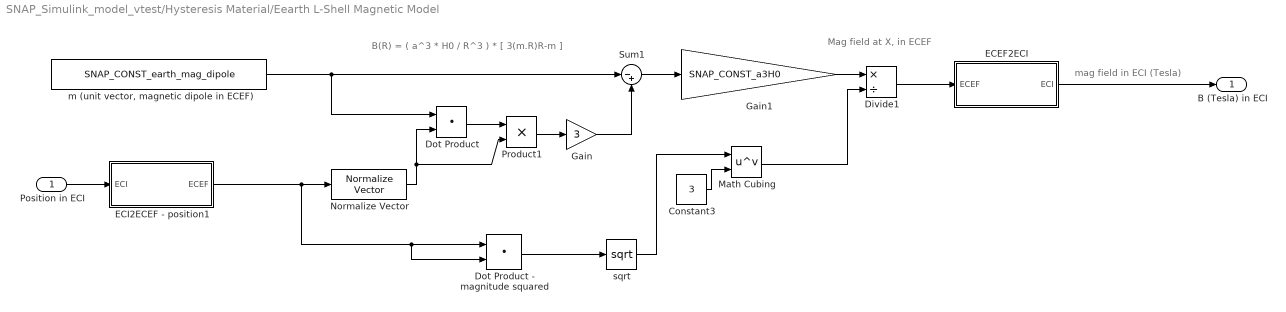
== system SNAP_Simulink_model_vtest/Hysteresis Material/Eearth L-Shell Magnetic Model ==
  note: B(R) = ( a^3 * H0 / R^3 ) * [ 3(m.R)R-m ]
  note: Mag field at X, in ECEF
  note: mag field in ECI (Tesla)
  Position in ECI : Inport
  Constant3 : Constant  Value=3
  Divide1 : Product  Inputs=*/
  Dot Product : DotProduct  InputSameDT=on  OutDataTypeStr=Inherit: Inherit via internal rule
  Dot Product - magnitude squared : DotProduct  InputSameDT=on  OutDataTypeStr=Inherit: Inherit via internal rule
  ECEF2ECI : Subsystem
  ECI2ECEF - position1 : Subsystem
  Gain : Gain  Gain=3
  Gain1 : Gain  Gain=SNAP_CONST_a3H0
  Math Cubing : Math  Operator=pow  SignedPower=on  SaturateOnIntegerOverflow=on
  Normalize Vector : vrlib/Utilities/Normalize Vector  maxzero=0
  Product1 : Product  RndMeth=Zero
  Sum1 : Sum  Inputs=|-+
  "m (unit vector, magnetic dipole in ECEF)" : Constant  Value=SNAP_CONST_earth_mag_dipole
  sqrt : Math  Operator=sqrt  SignedPower=on  SaturateOnIntegerOverflow=on
  B (Tesla) in ECI : Outport
  wires:
  "m (unit vector, magnetic dipole in ECEF)"/1 -> Dot Product/1, Sum1/1
  ECI2ECEF - position1/1(ECEF) -> Dot Product - magnitude squared/2, Dot Product - magnitude squared/1, Normalize Vector/1
  Dot Product/1 -> Product1/1
  Product1/1 -> Gain/1
  Gain/1 -> Sum1/2
  Sum1/1 -> Gain1/1
  Gain1/1 -> Divide1/1
  Dot Product - magnitude squared/1 -> sqrt/1
  sqrt/1 -> Math Cubing/1
  Constant3/1 -> Math Cubing/2
  Math Cubing/1 -> Divide1/2
  Divide1/1 -> ECEF2ECI/1(ECEF)
  Normalize Vector/1 -> Dot Product/2, Product1/2
  ECEF2ECI/1(ECI) -> B (Tesla) in ECI/1
  Position in ECI/1 -> ECI2ECEF - position1/1(ECI)

== system SNAP_Simulink_model_vtest/Hysteresis Material/Hysteresis Curve Model ==
  H : Inport
  Constant1 : Constant  Value=SNAP_Bs* 1e4
  Constant2 : Constant  Value=SNAP_Br* 1e4
  Constant3 : Constant  Value=SNAP_Hc
  Derivative : Derivative
  Gain : Gain  Gain=10000
  Gain2 : Gain  Gain=1/10000
  Hysteresis Model : MATLAB Function  TreatAsAtomicUnit=on
  Integrator : Integrator  InitialCondition=10000
  Rate Transition : RateTransition  Deterministic=off  OutPortSampleTimeOpt=Inherit  OutPortSampleTime=0.05
  Saturation1 : Saturate  UpperLimit=SNAP_Bs  LowerLimit=-SNAP_Bs
  B : Outport
  wires:
  Hysteresis Model/1(DBDT) -> Integrator/1
  Integrator/1 -> Gain2/1
  Gain/1 -> Hysteresis Model/1(B)
  Gain2/1 -> Saturation1/1
  Saturation1/1 -> Gain/1, B/1
  Rate Transition/1 -> Derivative/1, Hysteresis Model/2(H)
  Derivative/1 -> Hysteresis Model/3(DHDT)
  H/1 -> Rate Transition/1
  Constant1/1 -> Hysteresis Model/4(Bsx)
  Constant2/1 -> Hysteresis Model/5(Brx)
  Constant3/1 -> Hysteresis Model/6(Hcx)

== system SNAP_Simulink_model_vtest/Magnets/Eearth L-Shell Magnetic Model ==
  note: B(R) = ( a^3 * H0 / R^3 ) * [ 3(m.R)R-m ]
  note: Mag field at X, in ECEF
  note: mag field in ECI (Tesla)
  Position in ECI : Inport
  Constant3 : Constant  Value=3
  Divide1 : Product  Inputs=*/
  Dot Product : DotProduct  InputSameDT=on  OutDataTypeStr=Inherit: Inherit via internal rule
  Dot Product - magnitude squared : DotProduct  InputSameDT=on  OutDataTypeStr=Inherit: Inherit via internal rule
  ECEF2ECI : Subsystem
  ECI2ECEF - position1 : Subsystem
  Gain : Gain  Gain=3
  Gain1 : Gain  Gain=SNAP_CONST_a3H0
  Math Cubing : Math  Operator=pow  SignedPower=on  SaturateOnIntegerOverflow=on
  Normalize Vector : vrlib/Utilities/Normalize Vector  maxzero=0
  Product1 : Product  RndMeth=Zero
  Sum1 : Sum  Inputs=|-+
  "m (unit vector, magnetic dipole in ECEF)" : Constant  Value=SNAP_CONST_earth_mag_dipole
  sqrt : Math  Operator=sqrt  SignedPower=on  SaturateOnIntegerOverflow=on
  B (Tesla) in ECI : Outport
  wires:
  "m (unit vector, magnetic dipole in ECEF)"/1 -> Dot Product/1, Sum1/1
  ECI2ECEF - position1/1(ECEF) -> Dot Product - magnitude squared/2, Dot Product - magnitude squared/1, Normalize Vector/1
  Dot Product/1 -> Product1/1
  Product1/1 -> Gain/1
  Gain/1 -> Sum1/2
  Sum1/1 -> Gain1/1
  Gain1/1 -> Divide1/1
  Dot Product - magnitude squared/1 -> sqrt/1
  sqrt/1 -> Math Cubing/1
  Constant3/1 -> Math Cubing/2
  Math Cubing/1 -> Divide1/2
  Divide1/1 -> ECEF2ECI/1(ECEF)
  Normalize Vector/1 -> Dot Product/2, Product1/2
  ECEF2ECI/1(ECI) -> B (Tesla) in ECI/1
  Position in ECI/1 -> ECI2ECEF - position1/1(ECI)

== system SNAP_Simulink_model_vtest/ECI2ECEF - position/Direction Cosine Matrix ECI to ECEF1/Common Time Calculation ==
  JD : Inport
  deltaUT1 : Inport  Port=2
  deltaAT : Inport  Port=3
  Bias : Bias  Bias=32.184
  Bias1 : Bias  Bias=-51544.5
  Gain : Gain  Gain=1/36525
  Sum2 : Sum  Inputs=|++
  secGain : Gain  Gain=1/86400
  tTT : Outport
  ssUT : Outport  Port=2
  jdTT : Outport  Port=3
  wires:
  deltaAT/1 -> Bias/1
  Bias/1 -> secGain/1
  Bias1/1 -> Gain/1
  Gain/1 -> tTT/1
  deltaUT1/1 -> ssUT/1
  secGain/1 -> Sum2/2
  JD/1 -> Sum2/1
  Sum2/1 -> Bias1/1, jdTT/1

== system SNAP_Simulink_model_vtest/ECI2ECEF - position/Direction Cosine Matrix ECI to ECEF1/IAUReduction ==
  "[dX,dY]" : Inport
  "JD " : Inport  Port=2
  tTT : Inport  Port=3
  ssUT : Inport  Port=4
  jdTT : Inport  Port=5
  "[xp,yp]" : Inport  Port=6
  Additional Time Calculations : Subsystem
  Celestial motion of the CIP : Subsystem
  Earth Rotation : Subsystem
  Polar Motion : Subsystem
  Product : Product  Inputs=3  Multiplication=Matrix(*)
  Terminator : Terminator
  tTT1 : InportShadow  Port=3
  DCM : Outport
  wires:
  "[xp,yp]"/1 -> Polar Motion/2("[xp,yp]")
  Polar Motion/1(W) -> Product/1
  Celestial motion of the CIP/1(Q) -> Product/3
  jdTT/1 -> Terminator/1
  Product/1 -> DCM/1
  ssUT/1 -> Additional Time Calculations/1(ssUT)
  "JD "/1 -> Additional Time Calculations/2("JD ")
  tTT/1 -> Celestial motion of the CIP/2(tTT)
  "[dX,dY]"/1 -> Celestial motion of the CIP/1("[dX,dY]")
  Earth Rotation/1(R) -> Product/2
  tTT1/1 -> Polar Motion/1(tTT)
  Additional Time Calculations/1(jdElapsed) -> Earth Rotation/1(jdElapsed)
  Additional Time Calculations/2(jdFraction) -> Earth Rotation/2(jdFraction)

== system SNAP_Simulink_model_vtest/Hysteresis Material/Eearth L-Shell Magnetic Model/ECEF2ECI ==
  ECEF : Inport
  Constant1 : Constant  Value=[0 0]
  Constant3 : Constant  Value=SNAP_starting_ECI2ECEF_dcm
  Gain1 : Gain  Gain=-1
  Math Function2 : Math  Operator=transpose  SignedPower=on  SaturateOnIntegerOverflow=on
  Mux1 : Mux  Inputs=2
  Ramp2 : simulink/Sources/Ramp  slope="7.292115856e-5   %2*pi/(24*60*60)  %radians/second (one rotation per day )"  start=0  X0=0
  Rotation Angles to Direction Cosine Matrix1 : aerolibtransform2/Rotation Angles to Direction Cosine Matrix  rotationOrder=ZYX
      settings: SourceProductBaseCode=AE
  product 2 : Product  Multiplication=Matrix(*)  RndMeth=Zero
  product 4 : Product  Multiplication=Matrix(*)  RndMeth=Zero
  ECI : Outport
  wires:
  ECEF/1 -> product 4/1
  Ramp2/1 -> Gain1/1
  Gain1/1 -> Mux1/1
  Mux1/1 -> Rotation Angles to Direction Cosine Matrix1/1
  Constant1/1 -> Mux1/2
  product 2/1 -> Math Function2/1
  Rotation Angles to Direction Cosine Matrix1/1 -> product 2/2
  Constant3/1 -> product 2/1
  Math Function2/1 -> product 4/2
  product 4/1 -> ECI/1

== system SNAP_Simulink_model_vtest/Hysteresis Material/Eearth L-Shell Magnetic Model/ECI2ECEF - position1 ==
  ECI : Inport
  Constant : Constant  Value=[0 0]
  Constant2 : Constant  Value=SNAP_starting_ECI2ECEF_dcm
  Gain : Gain  Gain=-1
  Mux : Mux  Inputs=2
  Ramp1 : simulink/Sources/Ramp  slope="7.292115856e-5   %2*pi/(24*60*60)  %radians/second (one rotation per day )"  start=0  X0=0
  Rotation Angles to Direction Cosine Matrix : aerolibtransform2/Rotation Angles to Direction Cosine Matrix  rotationOrder=ZYX
      settings: SourceProductBaseCode=AE
  product 1 : Product  Multiplication=Matrix(*)  RndMeth=Zero
  product 2 : Product  Multiplication=Matrix(*)  RndMeth=Zero
  ECEF : Outport
  wires:
  product 2/1 -> ECEF/1
  ECI/1 -> product 2/1
  Ramp1/1 -> Gain/1
  Gain/1 -> Mux/1
  Mux/1 -> Rotation Angles to Direction Cosine Matrix/1
  Constant/1 -> Mux/2
  product 1/1 -> product 2/2
  Rotation Angles to Direction Cosine Matrix/1 -> product 1/2
  Constant2/1 -> product 1/1

== system SNAP_Simulink_model_vtest/Magnets/Eearth L-Shell Magnetic Model/ECEF2ECI ==
  ECEF : Inport
  Constant1 : Constant  Value=[0 0]
  Constant3 : Constant  Value=SNAP_starting_ECI2ECEF_dcm
  Gain1 : Gain  Gain=-1
  Math Function2 : Math  Operator=transpose  SignedPower=on  SaturateOnIntegerOverflow=on
  Mux1 : Mux  Inputs=2
  Ramp2 : simulink/Sources/Ramp  slope="7.292115856e-5   %2*pi/(24*60*60)  %radians/second (one rotation per day )"  start=0  X0=0
  Rotation Angles to Direction Cosine Matrix1 : aerolibtransform2/Rotation Angles to Direction Cosine Matrix  rotationOrder=ZYX
      settings: SourceProductBaseCode=AE
  product 2 : Product  Multiplication=Matrix(*)  RndMeth=Zero
  product 4 : Product  Multiplication=Matrix(*)  RndMeth=Zero
  ECI : Outport
  wires:
  ECEF/1 -> product 4/1
  Ramp2/1 -> Gain1/1
  Gain1/1 -> Mux1/1
  Mux1/1 -> Rotation Angles to Direction Cosine Matrix1/1
  Constant1/1 -> Mux1/2
  product 2/1 -> Math Function2/1
  Rotation Angles to Direction Cosine Matrix1/1 -> product 2/2
  Constant3/1 -> product 2/1
  Math Function2/1 -> product 4/2
  product 4/1 -> ECI/1

== system SNAP_Simulink_model_vtest/Magnets/Eearth L-Shell Magnetic Model/ECI2ECEF - position1 ==
  ECI : Inport
  Constant : Constant  Value=[0 0]
  Constant2 : Constant  Value=SNAP_starting_ECI2ECEF_dcm
  Gain : Gain  Gain=-1
  Mux : Mux  Inputs=2
  Ramp1 : simulink/Sources/Ramp  slope="7.292115856e-5   %2*pi/(24*60*60)  %radians/second (one rotation per day )"  start=0  X0=0
  Rotation Angles to Direction Cosine Matrix : aerolibtransform2/Rotation Angles to Direction Cosine Matrix  rotationOrder=ZYX
      settings: SourceProductBaseCode=AE
  product 1 : Product  Multiplication=Matrix(*)  RndMeth=Zero
  product 2 : Product  Multiplication=Matrix(*)  RndMeth=Zero
  ECEF : Outport
  wires:
  product 2/1 -> ECEF/1
  ECI/1 -> product 2/1
  Ramp1/1 -> Gain/1
  Gain/1 -> Mux/1
  Mux/1 -> Rotation Angles to Direction Cosine Matrix/1
  Constant/1 -> Mux/2
  product 1/1 -> product 2/2
  Rotation Angles to Direction Cosine Matrix/1 -> product 1/2
  Constant2/1 -> product 1/1

== system SNAP_Simulink_model_vtest/ECI2ECEF - position/Direction Cosine Matrix ECI to ECEF1/IAUReduction/Additional Time Calculations ==
  ssUT : Inport
  "JD " : Inport  Port=2
  Bias : Bias  Bias=-51544.5
  Constant : Constant
  Math Function : Math  Operator=mod  SignedPower=on  SaturateOnIntegerOverflow=on
  Sum : Sum  Inputs=|++
  gainVal : Gain  Gain=1/86400
  jdElapsed : Outport
  jdFraction : Outport  Port=2
  wires:
  gainVal/1 -> Sum/2
  ssUT/1 -> gainVal/1
  "JD "/1 -> Sum/1
  Sum/1 -> Bias/1  "jdUT1"
  Bias/1 -> Math Function/1, jdElapsed/1
  Math Function/1 -> jdFraction/1
  Constant/1 -> Math Function/2

== system SNAP_Simulink_model_vtest/ECI2ECEF - position/Direction Cosine Matrix ECI to ECEF1/IAUReduction/Celestial motion of the CIP ==
  "[dX,dY]" : Inport
  tTT : Inport  Port=2
  Lunisolar and planetary nutation : Subsystem
  P03 Precession : Subsystem
  Q : Outport
  wires:
  "[dX,dY]"/1 -> P03 Precession/1("[dX dY]")
  P03 Precession/1(Q) -> Q/1
  Lunisolar and planetary nutation/1(nutationV) -> P03 Precession/3(nutationV)
  tTT/1 -> P03 Precession/2(tTT), Lunisolar and planetary nutation/1(tTT)

== system SNAP_Simulink_model_vtest/ECI2ECEF - position/Direction Cosine Matrix ECI to ECEF1/IAUReduction/Earth Rotation ==
  jdElapsed : Inport
  jdFraction : Inport  Port=2
  Bias1 : Bias  Bias=0.7790572732640
  Constant : Constant  Value=2*pi
  Constant1 : Constant  Value=[0 0]
  Gain : Gain  Gain=0.00273781191135448
  Gain1 : Gain  Gain=2*pi
  Math Function : Math  Operator=mod  SignedPower=on  SaturateOnIntegerOverflow=on
  Mux : Mux  Inputs=2
  Rotation Angles to Direction Cosine Matrix : aerolibtransform2/Rotation Angles to Direction Cosine Matrix  rotationOrder=ZYX
      settings: SourceProductBaseCode=AE
  Sum : Sum  Inputs=|++
  R : Outport
  wires:
  Mux/1 -> Rotation Angles to Direction Cosine Matrix/1
  Rotation Angles to Direction Cosine Matrix/1 -> R/1
  Constant1/1 -> Mux/2
  Math Function/1 -> Mux/1  "thetaERA"
  Gain1/1 -> Math Function/1
  jdElapsed/1 -> Gain/1
  jdFraction/1 -> Bias1/1
  Constant/1 -> Math Function/2
  Bias1/1 -> Sum/1
  Gain/1 -> Sum/2
  Sum/1 -> Gain1/1

== system SNAP_Simulink_model_vtest/ECI2ECEF - position/Direction Cosine Matrix ECI to ECEF1/IAUReduction/Polar Motion ==
  tTT : Inport
  "[xp,yp]" : Inport  Port=2
  Angle Conversion : aerolibconvert2/Angle Conversion  IU=deg  OU=rad
  Demux : Demux  Outputs=2
  Gain : Gain  Gain=-0.000047/3600
  Gain1 : Gain  Gain=-1
  Mux : Mux  Inputs=3
  Rotation Angles to Direction Cosine Matrix : aerolibtransform2/Rotation Angles to Direction Cosine Matrix  rotationOrder=ZYX
      settings: SourceProductBaseCode=AE
  W : Outport
  wires:
  Rotation Angles to Direction Cosine Matrix/1 -> W/1
  Mux/1 -> Rotation Angles to Direction Cosine Matrix/1
  Gain/1 -> Angle Conversion/1
  tTT/1 -> Gain/1
  Angle Conversion/1 -> Mux/1  "sp"
  "[xp,yp]"/1 -> Gain1/1
  Gain1/1 -> Demux/1
  Demux/1 -> Mux/2
  Demux/2 -> Mux/3

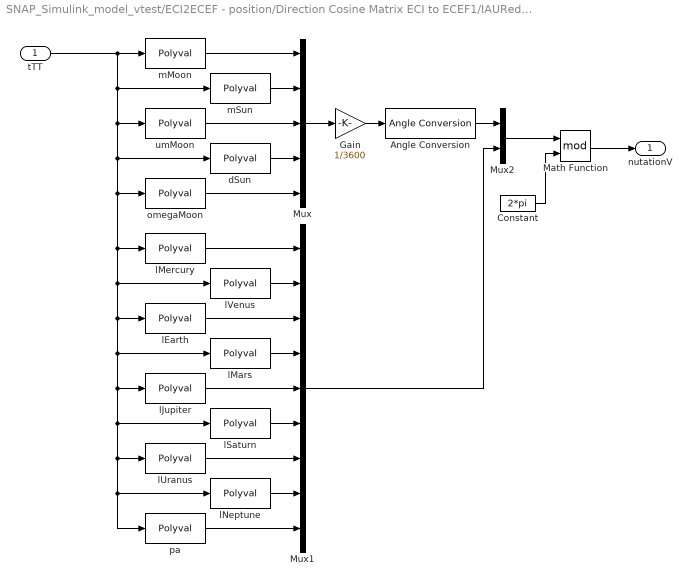
== system SNAP_Simulink_model_vtest/ECI2ECEF - position/Direction Cosine Matrix ECI to ECEF1/IAUReduction/Celestial motion of the CIP/Lunisolar and planetary nutation ==
  tTT : Inport
  Angle Conversion : aerolibconvert2/Angle Conversion  IU=deg  OU=rad
  Constant : Constant  Value=2*pi
  Gain : Gain  Gain=1/3600
  Math Function : Math  Operator=mod  SignedPower=on  SaturateOnIntegerOverflow=on
  Mux : Mux  Inputs=5
  Mux1 : Mux  Inputs=9
  Mux2 : Mux  Inputs=2
  dSun : Polyval  Coefs=[-0.00003169 0.006593 -6.3706 1602961601.2090 1072260.703692]
  lEarth : Polyval  Coefs=[628.3075849991 1.753470314]
  lJupiter : Polyval  Coefs=[52.9690962641 0.599546497]
  lMars : Polyval  Coefs=[334.06124267 6.203480913]
  lMercury : Polyval  Coefs=[2608.7903141574 4.402608842]
  lNeptune : Polyval  Coefs=[3.8133035638 5.311886287]
  lSaturn : Polyval  Coefs=[21.329910496 0.874016757]
  lUranus : Polyval  Coefs=[7.4781598567 5.481293872]
  lVenus : Polyval  Coefs=[1021.3285546211 3.176146697]
  mMoon : Polyval  Coefs=[-0.00024470 0.051635 31.8792 1717915923.2178 485868.249036]
  mSun : Polyval  Coefs=[-0.00001149 0.000136 -0.5532 129596581.0481 1287104.793048]
  omegaMoon : Polyval  Coefs=[-0.00005939 0.007702 7.4722 -6962890.5431 450160.398036]
  pa : Polyval  Coefs=[0.00000538691 0.02438175 0]
  umMoon : Polyval  Coefs=[0.00000417 -0.001037 -12.7512 1739527262.8478 335779.526232]
  nutationV : Outport
  wires:
  Mux1/1 -> Mux2/2
  pa/1 -> Mux1/9
  lNeptune/1 -> Mux1/8
  lUranus/1 -> Mux1/7
  lSaturn/1 -> Mux1/6
  lJupiter/1 -> Mux1/5
  lMars/1 -> Mux1/4
  Math Function/1 -> nutationV/1
  Constant/1 -> Math Function/2
  Mux2/1 -> Math Function/1
  Angle Conversion/1 -> Mux2/1
  lEarth/1 -> Mux1/3
  lVenus/1 -> Mux1/2
  lMercury/1 -> Mux1/1
  Gain/1 -> Angle Conversion/1
  Mux/1 -> Gain/1
  omegaMoon/1 -> Mux/5
  dSun/1 -> Mux/4
  umMoon/1 -> Mux/3
  mSun/1 -> Mux/2
  mMoon/1 -> Mux/1
  tTT/1 -> mMoon/1, mSun/1, umMoon/1, omegaMoon/1, lMercury/1, lEarth/1, lMars/1, lJupiter/1, lSaturn/1, lUranus/1, lNeptune/1, pa/1, lVenus/1, dSun/1

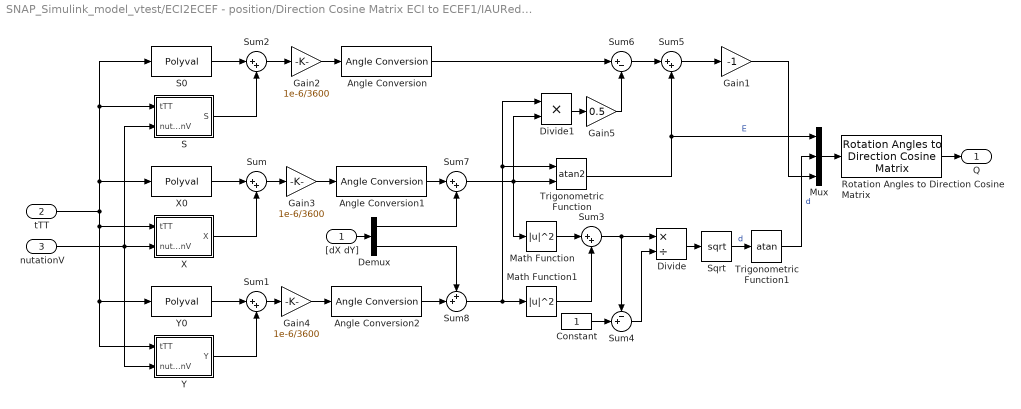
== system SNAP_Simulink_model_vtest/ECI2ECEF - position/Direction Cosine Matrix ECI to ECEF1/IAUReduction/Celestial motion of the CIP/P03 Precession ==
  "[dX dY]" : Inport
  tTT : Inport  Port=2
  nutationV : Inport  Port=3
  Angle Conversion : aerolibconvert2/Angle Conversion  IU=deg  OU=rad
  Angle Conversion1 : aerolibconvert2/Angle Conversion  IU=deg  OU=rad
  Angle Conversion2 : aerolibconvert2/Angle Conversion  IU=deg  OU=rad
  Constant : Constant
  Demux : Demux  Outputs=2
  Divide : Product  Inputs=*/
  Divide1 : Product  Inputs=**
  Gain1 : Gain  Gain=-1
  Gain2 : Gain  Gain=1e-6/3600
  Gain3 : Gain  Gain=1e-6/3600
  Gain4 : Gain  Gain=1e-6/3600
  Gain5 : Gain  Gain=0.5
  Math Function : Math  Operator=magnitude^2  SignedPower=on  SaturateOnIntegerOverflow=on
  Math Function1 : Math  Operator=magnitude^2  SignedPower=on  SaturateOnIntegerOverflow=on
  Mux : Mux  Inputs=3
  Rotation Angles to Direction Cosine Matrix : aerolibtransform2/Rotation Angles to Direction Cosine Matrix  rotationOrder=ZYZ
      settings: SourceProductBaseCode=AE
  S : Subsystem
  S0 : Polyval  Coefs="[15.62 27.98 -72574.11 -122.68 3808.65  94]"
  Sqrt : Sqrt  SaturateOnIntegerOverflow=on
  Sum{,1..3,5,7} (6 alike) : Sum  Inputs=|++
  Sum4 : Sum  Inputs=-+|
  Sum6 : Sum  Inputs=|+-
  Sum8 : Sum  Inputs=++|
  Trigonometric Function : Trigonometry  Operator=atan2
  Trigonometric Function1 : Trigonometry  Operator=atan
  X : Subsystem
  X0 : Polyval  Coefs=[5.9285 7.578 -198618.34 -429782.9 2004191898 -16617]
  Y : Subsystem
  Y0 : Polyval  Coefs=[0.1358 1112.526 1900.59 -22407274.7 -25896 -6951]
  Q : Outport
  wires:
  Trigonometric Function1/1 -> Mux/2  "d"
  Sqrt/1 -> Trigonometric Function1/1  "d"
  S/1(S) -> Sum2/2
  Y/1(Y) -> Sum1/2
  "[dX dY]"/1 -> Demux/1
  Sum6/1 -> Sum5/1
  Gain5/1 -> Sum6/2
  Divide1/1 -> Gain5/1
  Angle Conversion/1 -> Sum6/1
  Sum8/1 -> Math Function1/1, Trigonometric Function/1, Divide1/1
  Gain4/1 -> Angle Conversion2/1
  Gain3/1 -> Angle Conversion1/1
  Sum7/1 -> Trigonometric Function/2, Math Function/1, Divide1/2
  Gain2/1 -> Angle Conversion/1
  Rotation Angles to Direction Cosine Matrix/1 -> Q/1
  Mux/1 -> Rotation Angles to Direction Cosine Matrix/1
  Sum2/1 -> Gain2/1
  Trigonometric Function/1 -> Mux/1, Sum5/2  "E"
  Divide/1 -> Sqrt/1
  Sum4/1 -> Divide/2
  Constant/1 -> Sum4/2
  Sum3/1 -> Divide/1, Sum4/1
  Math Function1/1 -> Sum3/2
  Math Function/1 -> Sum3/1
  Sum/1 -> Gain3/1
  Sum1/1 -> Gain4/1
  S0/1 -> Sum2/1
  tTT/1 -> Y0/1, Y/1(tTT), X/1(tTT), S0/1, S/1(tTT), X0/1
  nutationV/1 -> S/2(nutationV), X/2(nutationV), Y/2(nutationV)
  Sum5/1 -> Gain1/1
  Gain1/1 -> Mux/3
  Y0/1 -> Sum1/1
  X/1(X) -> Sum/2
  X0/1 -> Sum/1
  Angle Conversion2/1 -> Sum8/2
  Demux/2 -> Sum8/1
  Angle Conversion1/1 -> Sum7/1
  Demux/1 -> Sum7/2

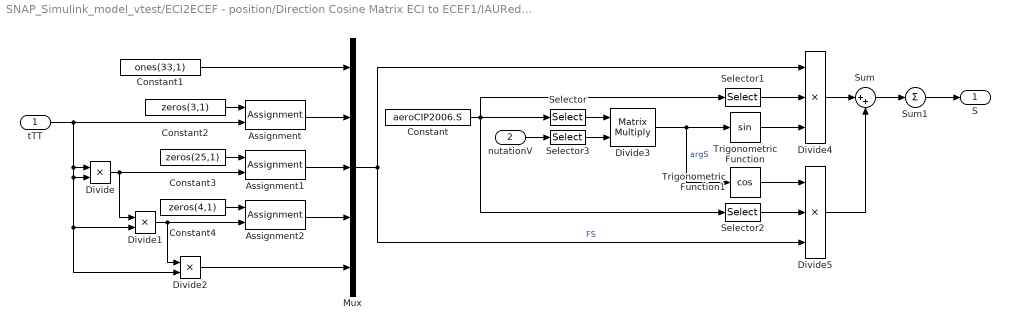
== system SNAP_Simulink_model_vtest/ECI2ECEF - position/Direction Cosine Matrix ECI to ECEF1/IAUReduction/Celestial motion of the CIP/P03 Precession/S ==
  tTT : Inport
  nutationV : Inport  Port=2
  Assignment : Assignment  IndexOptions=Assign all  Indices=1  OutputSizes=1
  Assignment1 : Assignment  IndexOptions=Assign all  Indices=1  OutputSizes=1
  Assignment2 : Assignment  IndexOptions=Assign all  Indices=1  OutputSizes=1
  Constant : Constant  Value=aeroCIP2006.S
  Constant1 : Constant  Value=ones(33,1)
  Constant2 : Constant  Value=zeros(3,1)
  Constant3 : Constant  Value=zeros(25,1)
  Constant4 : Constant  Value=zeros(4,1)
  Divide : Product  Inputs=**
  Divide1 : Product  Inputs=**
  Divide2 : Product  Inputs=**
  Divide3 : Product  Inputs=**  Multiplication=Matrix(*)
  Divide4 : Product  Inputs=***
  Divide5 : Product  Inputs=***
  Mux : Mux  Inputs=5
  Selector : Selector  NumberOfDimensions=2  InputPortWidth=3  IndexOptions=Select all,Index vector (dialog)  Indices=[1 3],[4 5 6 7 8 9 10 11]  OutputSizes=1,11
  Selector1 : Selector  NumberOfDimensions=2  InputPortWidth=3  IndexOptions=Select all,Index vector (dialog)  Indices=[1 3],2  OutputSizes=1,14
  Selector2 : Selector  NumberOfDimensions=2  InputPortWidth=3  IndexOptions=Select all,Index vector (dialog)  Indices=[1 3],3  OutputSizes=1,14
  Selector3 : Selector  InputPortWidth=14  IndexOptions=Index vector (dialog)  Indices=[1 2 3 4 5 7 8 14]  OutputSizes=1
  Sum : Sum  Inputs=|++
  Sum1 : Sum  Inputs=|+|
  Trigonometric Function : Trigonometry
  Trigonometric Function1 : Trigonometry  Operator=cos
  S : Outport
  wires:
  Constant1/1 -> Mux/1
  Assignment/1 -> Mux/2
  Assignment1/1 -> Mux/3
  Assignment2/1 -> Mux/4
  Divide2/1 -> Mux/5
  Sum1/1 -> S/1
  Sum/1 -> Sum1/1
  Divide5/1 -> Sum/2
  Divide4/1 -> Sum/1
  Mux/1 -> Divide5/3, Divide4/1  "FS"
  Selector2/1 -> Divide5/2
  Trigonometric Function1/1 -> Divide5/1
  Selector1/1 -> Divide4/2
  Trigonometric Function/1 -> Divide4/3
  Divide3/1 -> Trigonometric Function/1, Trigonometric Function1/1  "argS"
  Constant/1 -> Selector2/1, Selector1/1, Selector/1
  Divide/1 -> Assignment1/2, Divide1/1
  Divide1/1 -> Assignment2/2, Divide2/1
  Constant4/1 -> Assignment2/1
  Constant3/1 -> Assignment1/1
  tTT/1 -> Assignment/2, Divide/1, Divide/2, Divide1/2, Divide2/2
  Constant2/1 -> Assignment/1
  nutationV/1 -> Selector3/1
  Selector3/1 -> Divide3/2
  Selector/1 -> Divide3/1
